simulink model "nonliner_saturation_2"  (R2019a)
settings: Solver=VariableStepAuto  StartTime=0.0  StopTime=500  RelTol=1e-3
libraries: simulink x2
settings Model: Creator=Mohamed Nofal  LastModifiedBy=Mohamed Nofal

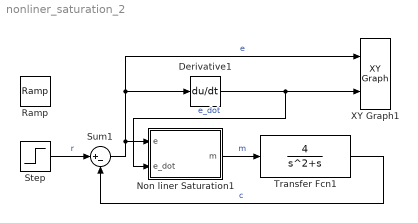
== system nonliner_saturation_2 ==
  Derivative1 : Derivative
  Non liner Saturation1 : MATLAB Function  TreatAsAtomicUnit=on
  Ramp : simulink/Sources/Ramp  slope=0.7  start=0  InitialOutput=0
  Step : Step  SampleTime=0
  Sum1 : Sum  Inputs=|+-
  Transfer Fcn1 : TransferFcn  Numerator=[4]  Denominator=[1,1,0]
  XY Graph1 : simulink/Sinks/XY Graph  xmin=-1  xmax=1  ymin=-1  ymax=1  st=.1
  wires:
  Non liner Saturation1/1(m) -> Transfer Fcn1/1  "m"
  Sum1/1 -> Non liner Saturation1/1(e), XY Graph1/1, Derivative1/1  "e"
  Transfer Fcn1/1 -> Sum1/2  "c"
  Step/1 -> Sum1/1  "r"
  Derivative1/1 -> Non liner Saturation1/2(e_dot), XY Graph1/2  "e_dot"

== matlab function nonliner_saturation_2/Non liner Saturation1 ==
  data: e input; m output; e_dot input
function m = fcn(e,e_dot)
if e_dot >0
    if e<-0.1
        m=-0.2;
    elseif e>0.2
        m=0.2;
    else 
        m=0;
    end
else
    if e<-0.2
        m=-0.2;
    elseif e>0.1
        m=0.2;
    else 
        m=0;
    end
end
m=m ;
